simulink model "modelStaticna"  (R2020b)
settings: Solver=VariableStepAuto  StartTime=0.0  StopTime=140  RelTol=1e-3
values from neighbouring files (symbols this model uses):
  f0 = 0.105    [Linear.m]    (also in NelinearniModel.m; Optimizacija.m; modelrez.mat)
  J = ro_d*((1/3)*l1*(r1^2 - r1*r2 + r2^2) + l2*((l2^2/3) + r2^2)) + mm*lm^2 + mu1*lu1^2 + mu2*lu2^2    (= 0.0484953922533)    [Linear.m]    (also in NelinearniModel.m; Optimizacija.m; modelrez.mat)
  k1 = g*(ro_d*(((r2^2)/2 - (r1^2)/2)) + mu1*lu1 - mm*lm)    (= -0.66893409)    [Linear.m]    (also in NelinearniModel.m = -0.62324; Optimizacija.m; modelrez.mat; objectiveFunction.m = params(1))
  k2 = ro_d*g*l2d    [Linear.m]    (also in NelinearniModel.m = 0.22329; Optimizacija.m = ro_d * g * l2d; modelrez.mat = 0.297959350185; objectiveFunction.m = params(2))
  k3 = mu2*g*lu2    (= 0.0565056)    [Linear.m]    (also in NelinearniModel.m = 0.085677; Optimizacija.m; modelrez.mat)
  lm = 0.38    [Linear.m]    (also in NelinearniModel.m; Optimizacija.m; modelrez.mat)
  psi_1 = deg2rad(17.74)    [Linear.m]    (also in NelinearniModel.m; Optimizacija.m; modelrez.mat = 0.309621409304)
  psi_2 = deg2rad(33.62)    [Linear.m]    (also in NelinearniModel.m; Optimizacija.m; modelrez.mat = 0.58677969452)
undefined symbols (not defined in the file or in its folder): K1
settings Model: Creator=Acer  LastModifiedBy=Acer

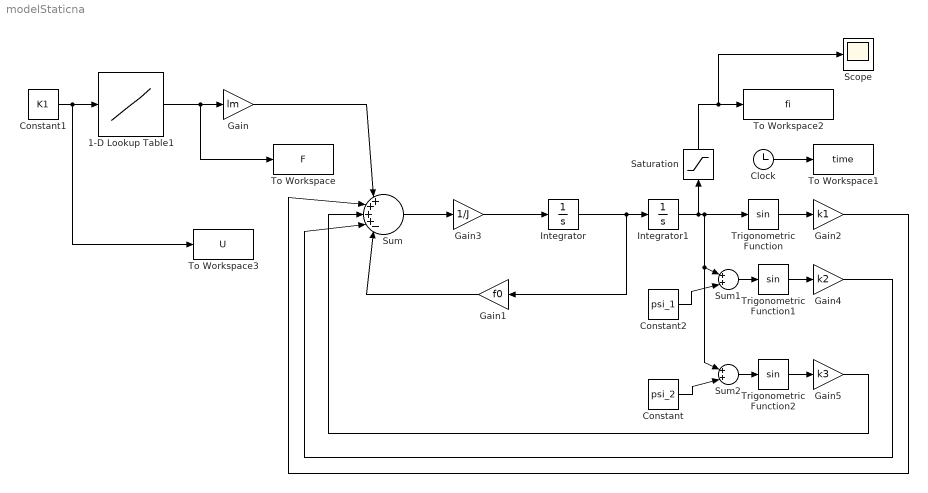
== system modelStaticna ==
  1-D Lookup Table1 : Lookup_n-D  NumberOfTableDimensions=1  BreakpointsForDimension1=[0,4.6, 4.7, 5, 5.5, 6, 7, 7.5, 8, 8.5, 10]  Table=[0,0,0.10984,0.21163,0.38639,0.54977,0.9284,0.9284,0.9284, 0.9284,0.9284]  InternalRulePriority=Speed  RndMeth=Simplest  InputSameDT=on
  Clock : Clock
  Constant : Constant  Value=psi_2
  Constant1 : Constant  Value=K1
  Constant2 : Constant  Value=psi_1
  Gain : Gain  Gain=lm
  Gain1 : Gain  Gain=f0
  Gain2 : Gain  Gain=k1
  Gain3 : Gain  Gain=1/J
  Gain4 : Gain  Gain=k2
  Gain5 : Gain  Gain=k3
  Integrator : Integrator
  Integrator1 : Integrator
  Saturation : Saturate  UpperLimit=3.0717  LowerLimit=0
  Scope : Scope
  Sum : Sum  Inputs=|++++-|
  Sum1 : Sum  Inputs=|++|
  Sum2 : Sum  Inputs=|++|
  To Workspace : ToWorkspace  VariableName=F  SampleTime=-1
  To Workspace1 : ToWorkspace  VariableName=time  SampleTime=-1
  To Workspace2 : ToWorkspace  VariableName=fi  SaveFormat=Timeseries  SampleTime=0.1
  To Workspace3 : ToWorkspace  VariableName=U  SampleTime=-1
  Trigonometric Function : Trigonometry
  Trigonometric Function1 : Trigonometry
  Trigonometric Function2 : Trigonometry
  wires:
  Gain4/1 -> Sum/4
  Sum2/1 -> Trigonometric Function2/1
  Integrator/1 -> Integrator1/1, Gain1/1
  Gain1/1 -> Sum/5
  Constant2/1 -> Sum1/2
  Trigonometric Function2/1 -> Gain5/1
  Trigonometric Function/1 -> Gain2/1
  Gain/1 -> Sum/1
  Gain2/1 -> Sum/2
  Constant/1 -> Sum2/2
  Sum/1 -> Gain3/1
  Gain5/1 -> Sum/3
  Constant1/1 -> 1-D Lookup Table1/1, To Workspace3/1
  Gain3/1 -> Integrator/1
  1-D Lookup Table1/1 -> To Workspace/1, Gain/1
  Trigonometric Function1/1 -> Gain4/1
  Sum1/1 -> Trigonometric Function1/1
  Integrator1/1 -> Trigonometric Function/1, Sum2/1, Sum1/1, Saturation/1
  Clock/1 -> To Workspace1/1
  Saturation/1 -> To Workspace2/1, Scope/1
